simulink model "ParityChecker"  (R2025b)
settings: Solver=FixedStepDiscrete  StartTime=0.0  StopTime=Inf  RelTol=1e-3
settings Model: Creator=Soochan Kim  LastModifiedBy=Soochan Kim
settings OptimizationCC: BlockReduction=off  ConditionallyExecuteInputs=off  DefaultParameterBehavior=Inlined
settings DebuggingCC: AlgebraicLoopMsg=error
settings HardwareCC: ProdBitPerPointer=32.0  ProdBitPerSizeT=32.0  ProdBitPerPtrDiffT=32.0  ProdLargestAtomicFloat=None  ProdIntDivRoundTo=Undefined  ProdEndianess=Unspecified  ProdWordSize=32.0  ProdHWDeviceType=ASIC/FPGA->ASIC/FPGA  TargetBitPerPointer=64.0  TargetBitPerSizeT=64.0  TargetBitPerPtrDiffT=64.0  TargetLongLongMode=on  TargetIntDivRoundTo=Zero  TargetEndianess=LittleEndian  TargetWordSize=64.0  TargetHWDeviceType=Custom Processor->MATLAB Host Computer  ProdEqTarget=off

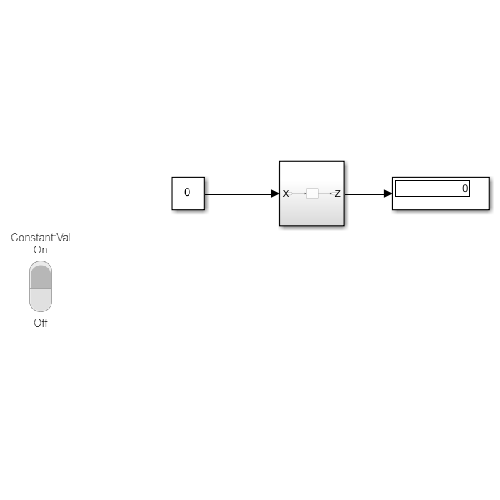
[thumbnail: Simulink's stored preview of the top-level diagram]
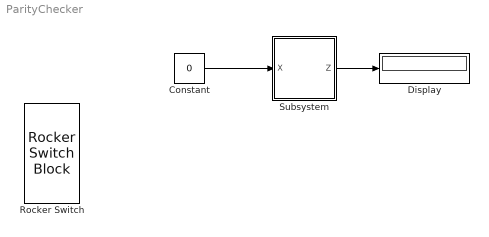
== system ParityChecker ==
  Constant : Constant  Value=0  OutDataTypeStr=boolean
  Display : Display
  Rocker Switch : RockerSwitchBlock
  Subsystem : Subsystem
  wires:
  Constant/1 -> Subsystem/1(X)
  Subsystem/1(Z) -> Display/1

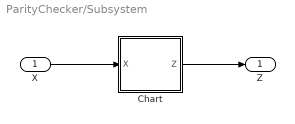
== system ParityChecker/Subsystem ==
  X : Inport
  Chart : Stateflow chart  TreatAsAtomicUnit=on
  Z : Outport
  wires:
  X/1 -> Chart/1(X)
  Chart/1(Z) -> Z/1

== stateflow chart ParityChecker/Subsystem/Chart ==
  settings: stateMachineType=MOORE_MACHINE  executeAtInitialization=1  initializeOutput=1
  state S0
    Z = false;
  state S1
    Z = true;
  (default) -> S0
  S0 -> S1 : [X==1]
  S1 -> S0 : [X==1]
  data: Z output boolean; X input boolean
